simulink model "two_wires"  (R2021b)
settings: Solver=VariableStepAuto  StartTime=0.0  StopTime=5  FixedStep=0.1  RelTol=1e-3
settings Model: Creator=teja  LastModifiedBy=teja

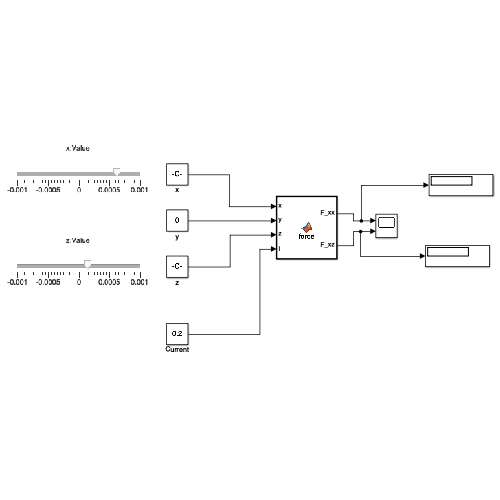
[thumbnail: Simulink's stored preview of the top-level diagram]
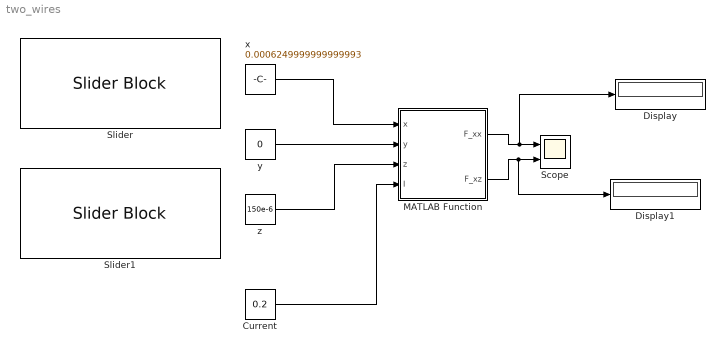
== system two_wires ==
  Current : Constant  Value=0.2
  Display : Display
  Display1 : Display
  MATLAB Function : MATLAB Function  TreatAsAtomicUnit=on
  Scope : Scope  NumInputPorts=2
  Slider : SliderBlock  ScaleMin=-1000e-6  ScaleMax=1000e-6
  Slider1 : SliderBlock  ScaleMin=-1000e-6  ScaleMax=1000e-6
  x : Constant  Value=0.0006249999999999993
  y : Constant  Value=0
  z : Constant  Value=150e-6
  wires:
  MATLAB Function/1(F_xx) -> Display/1, Scope/1
  MATLAB Function/2(F_xz) -> Display1/1, Scope/2
  x/1 -> MATLAB Function/1(x)
  y/1 -> MATLAB Function/2(y)
  z/1 -> MATLAB Function/3(z)
  Current/1 -> MATLAB Function/4(I)

== matlab function two_wires/MATLAB Function ==
  data: x input; F_xx output; F_xz output; y input; z input; I input
function [F_xx, F_xz] = force(x, y, z, I)

g = 200e-6;     %Coil spaxing               - ONLY g is different and y1_1 like parameters
m0 = 4*pi*1e-7;
radius = 3e-3;%m
height = 1e-3;%m
Magentization = 1.45; %T
vol_cy = pi*radius^2*height; %If Object is Cylinder, vol in m^3
y1_1 = g;
y2_1 = -g;
a_xp_1 = g;          %Distanxe of xoil from (0,0)

k_yp_1 = 1/(4*pi*((a_xp_1-x)^2+z^2));
k_1yp_1 = (y2_1-y)/((y2_1-y)^2+(a_xp_1-x)^2+z^2)^0.5;
k_2yp_1 = (y1_1-y)/((y1_1-y)^2+(a_xp_1-x)^2+z^2)^0.5;

a_xn_1 = -g;
k_yn_1 = 1/(4*pi*((a_xn_1-x)^2+z^2));
k_1yn_1 = (y2_1-y)/((y2_1-y)^2+(a_xn_1-x)^2+z^2)^0.5;
k_2yn_1 = (y1_1-y)/((y1_1-y)^2+(a_xn_1-x)^2+z^2)^0.5;

%--------%--------%--------%--------%--------%--------%--------%----------
%2nd Proof - Gradient
%-%--------%--------%--------%--------%--------%--------%--------%--------
k_1yp_3 = (y2_1-y)/((y2_1-y)^2+(a_xp_1-x)^2+z^2)^1.5;
k_2yp_3 = (y1_1-y)/((y1_1-y)^2+(a_xp_1-x)^2+z^2)^1.5;
k_1yn_3 = (y2_1-y)/((y2_1-y)^2+(a_xn_1-x)^2+z^2)^1.5;
k_2yn_3 = (y1_1-y)/((y1_1-y)^2+(a_xn_1-x)^2+z^2)^1.5;
hp = -(z*k_yp_1*(a_xp_1-x))*I*m0;
hp_1 = (k_yp_1*(k_1yp_1 - k_2yp_1))*2*4*pi;
hp_2 = k_1yp_3 - k_2yp_3;
df_xx = hp*(hp_1 + hp_2);

hp_z = (k_yp_1)*I*m0;
hp_z1 = (k_1yp_1 - k_2yp_1)*(-1);
hp_z2 = (k_yp_1*(k_1yp_1 - k_2yp_1)*(z^2))*4*pi*2;
hp_z3 = (k_1yp_3 - k_2yp_3)*(z^2);
df_xz = hp_z*(hp_z1 + hp_z2 + hp_z3);

hn = -(z*k_yn_1*(a_xn_1-x))*I*m0;
hn_1 = (k_yn_1*(k_1yn_1 - k_2yn_1))*2*4*pi;
hn_2 = k_1yn_3 - k_2yn_3;
df_xx_n = hn*(hn_1 + hn_2);

hn_z = (k_yn_1)*I*m0;
hn_z1 = (k_1yn_1 - k_2yn_1)*(-1);
hn_z2 = (k_yn_1*(k_1yn_1 - k_2yn_1)*(z^2))*4*pi*2;
hn_z3 = (k_1yn_3 - k_2yn_3)*(z^2);
df_xz_n = hn_z*(hn_z1 + hn_z2 + hn_z3);

%--------%--------%--------%--------%--------%--------%--------%----------
%3rd Proof - Force
%-%--------%--------%--------%--------%--------%--------%--------%--------
F_xx = vol_cy * Magentization* (df_xx + df_xx_n)/m0;
F_xz = vol_cy * Magentization* (df_xz + df_xz_n)/m0;
end
